simulink model "SDT505SimpleMotorModelLegDemux"  (R2022b)
settings: Solver=VariableStepAuto  StartTime=0.0  StopTime=10.0  RelTol=1e-3
settings Model: Creator=mjbou  LastModifiedBy=mjbou

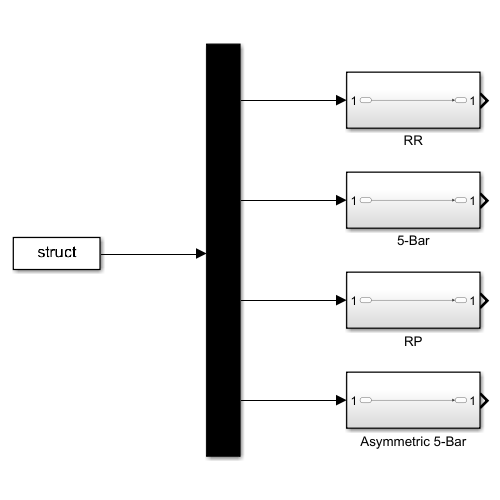
[thumbnail: Simulink's stored preview of the top-level diagram]
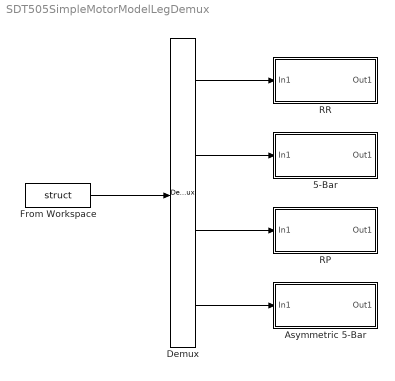
== system SDT505SimpleMotorModelLegDemux ==
  5-Bar : Subsystem
  Asymmetric 5-Bar : Subsystem
  Demux : Demux
  From Workspace : FromWorkspace  VariableName=struct
  RP : Subsystem
  RR : Subsystem
  wires:
  From Workspace/1 -> Demux/1
  Demux/1 -> RR/1(In1)
  Demux/3 -> RP/1(In1)
  Demux/2 -> 5-Bar/1(In1)
  Demux/4 -> Asymmetric 5-Bar/1(In1)

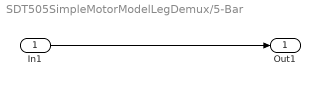
== system SDT505SimpleMotorModelLegDemux/5-Bar ==
  In1 : Inport
  Out1 : Outport
  wires:
  In1/1 -> Out1/1

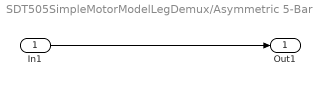
== system SDT505SimpleMotorModelLegDemux/Asymmetric 5-Bar ==
  In1 : Inport
  Out1 : Outport
  wires:
  In1/1 -> Out1/1

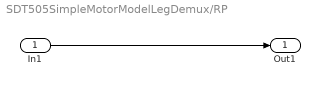
== system SDT505SimpleMotorModelLegDemux/RP ==
  In1 : Inport
  Out1 : Outport
  wires:
  In1/1 -> Out1/1

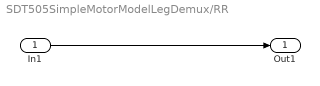
== system SDT505SimpleMotorModelLegDemux/RR ==
  In1 : Inport
  Out1 : Outport
  wires:
  In1/1 -> Out1/1
